simulink model "lab01_2"  (R2025a)
settings: Solver=VariableStepAuto  StartTime=0.0  StopTime=50  RelTol=1e-3
libraries: slctrl_linear x1
settings Model: Creator=grigorijtomczuk  LastModifiedBy=grigorijtomczuk

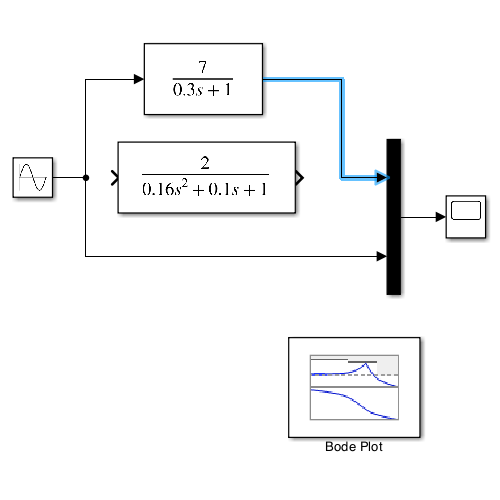
[thumbnail: Simulink's stored preview of the top-level diagram]
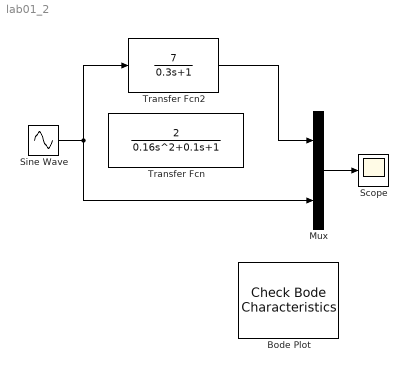
== system lab01_2 ==
  Bode Plot : slctrl_linear/Check Bode  Characteristics  InstantiateOnLoad=on  SaveOperatingPoints=off  LinearizationIOs={'/Transfer Fcn', 1, 'out', 'on', '';'/Sine Wave', 1, 'in', 'off', '';'/Transfer Fcn2', 1, 'out', 'on', ''}  LinearizeAt=SnapshotTimes  SnapshotTimes=[0]  TriggerType=rising  SampleTime=auto  RateConversionMethod=zoh  PreWarpFreq=10  UseExactDelayModel=off  UseFullBlockNameLabels=off  UseBusSignalLabels=off  enabled=on  stopWhenAssertionFail=off  export=off  ViewDlgPos=[567 157 778 599]  OpenViewOnLoad=on  LaunchViewOnOpen=off  FrequencyUnits=rad/s  MagnitudeUnits=dB  PhaseUnits=deg  TimeUnits=seconds  EnableUpperBound=off  UpperBoundFrequencies=[]  UpperBoundMagnitudes=[]  EnableLowerBound=off  LowerBoundFrequencies=[]  LowerBoundMagnitudes=[]
      settings: LibrarySourceBlock=slctrlblks/Linear Analysis Plots/Bode Plot  SaveToWorkspace=off  SaveName=sys
  Mux : Mux  Inputs=2
  Scope : Scope
      settings: ActiveDisplayYMinimum=-3.0215809559451112  ActiveDisplayYMaximum=3.3843529814382425
  Sine Wave : Sin  SampleTime=0
  Transfer Fcn : TransferFcn  Numerator=[2]  Denominator=[0.16 0.1 1]
  Transfer Fcn2 : TransferFcn  Numerator=[7]  Denominator=[0.3 1]
  wires:
  Sine Wave/1 -> Transfer Fcn2/1, Mux/2
  Transfer Fcn2/1 -> Mux/1
  Mux/1 -> Scope/1
